simulink model "Compass_fn"  (Simulink 7.0)
settings: Solver=ode45  StartTime=0.0  StopTime=10.0  RelTol=1e-3
settings Model: Creator=volgy  LastModifiedBy=Nag

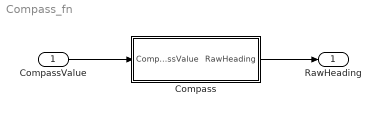
== system Compass_fn ==
  CompassValue : Inport  OutDataType=sfix(16)  OutScaling=2^0
  Compass : Subsystem
  RawHeading : Outport  OutDataType=sfix(16)  OutScaling=2^0
  wires:
  CompassValue/1 -> Compass/1(CompassValue)
  Compass/1(RawHeading) -> RawHeading/1

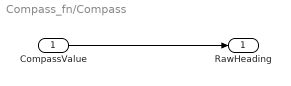
== system Compass_fn/Compass ==
  CompassValue : Inport  OutDataType=sfix(16)  OutScaling=2^0
  RawHeading : Outport  OutDataType=sfix(16)  OutScaling=2^0
  wires:
  CompassValue/1 -> RawHeading/1
